simulink model "TrajectoryGeneratorASYNC"  (R2020a)
settings: Solver=FixedStepAuto  StartTime=0.0  StopTime=inf  RelTol=1e-3
model workspace (MAT data in the model file):
  SL_ROS_VariableLengthArrays_MaxSizes.CommonInfo.ArrayTruncateAction = 'EmitWarning'
  SL_ROS_VariableLengthArrays_MaxSizes.MsgTypeMap = containers.Map
  SL_ROS_VariableLengthArrays_MaxSizes.MsgTypeMap.serialization.keys = {}
  SL_ROS_VariableLengthArrays_MaxSizes.MsgTypeMap.serialization.values = {}
  SL_ROS_VariableLengthArrays_MaxSizes.MsgTypeMap.serialization.uniformity = 0
  SL_ROS_VariableLengthArrays_MaxSizes.MsgTypeMap.serialization.keyType = 'char'
  SL_ROS_VariableLengthArrays_MaxSizes.MsgTypeMap.serialization.valueType = 'any'
settings Model: Creator=Lamarre  LastModifiedBy=alexemdesgagne
settings DataIOCC: SaveOutput=off  SaveTime=off
settings OptimizationCC: EnhancedBackFolding=on  PassReuseOutputArgsAs=Individual arguments  ZeroExternalMemoryAtStartup=off  ZeroInternalMemoryAtStartup=off  MaxStackSize=64  OptimizeBlockOrder=speed  DifferentSizesBufferReuse=on  OptimizationCustomize=off  EfficientTunableParamExpr=on
settings DebuggingCC: ParameterTunabilityLossMsg=error  FcnCallInpInsideContextMsg=warning  UnderSpecifiedDimensionMsg=warning
settings HardwareCC: ProdBitPerLong=64  ProdHWDeviceType=Intel->x86-64 (Linux 64)
settings ModelReferenceCC: ModelReferenceNumInstancesAllowed=Single
settings SFSimCC: MATLABDynamicMemAlloc=off
settings RTWCC: SystemTargetFile=ert.tlc  HardwareBoard=Robot Operating System (ROS)  TemplateMakefile=ert_default_tmf  Toolchain=Catkin  BuildConfiguration=Faster Runs  TargetLang=C++
settings CodeAppCC: ForceParamTrailComments=on  IgnoreCustomStorageClasses=off  OperatorAnnotations=on  SimulinkDataObjDesc=on  SFDataObjDesc=on  InsertBlockDesc=on
settings ERTTargetCC: SuppressErrorStatus=on  SupportVariableSizeSignals=on  MultiInstanceErrorCode=Warning  RootIOFormat=Structure reference

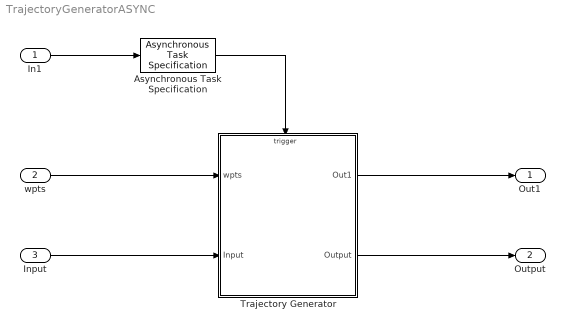
== system TrajectoryGeneratorASYNC ==
  In1 : Inport  OutDataTypeStr=boolean  PortDimensions=1  OutputFunctionCall=on
  wpts : Inport  Port=2  OutDataTypeStr=double  PortDimensions=[20 7]
  Input : Inport  Port=3  OutDataTypeStr=double  PortDimensions=[1 1]
  Asynchronous Task Specification : AsynchronousTaskSpecification
  Trajectory Generator : Subsystem  TreatAsAtomicUnit=on
  Out1 : Outport  OutDataTypeStr=double  PortDimensions=[1000 13]
  Output : Outport  Port=2  OutDataTypeStr=double  PortDimensions=[1 2]
  wires:
  Trajectory Generator/2(Output) -> Output/1
  In1/1 -> Asynchronous Task Specification/1
  Asynchronous Task Specification/1 -> Trajectory Generator/Trigger
  wpts/1 -> Trajectory Generator/1(wpts)
  Trajectory Generator/1(Out1) -> Out1/1
  Input/1 -> Trajectory Generator/2(Input)

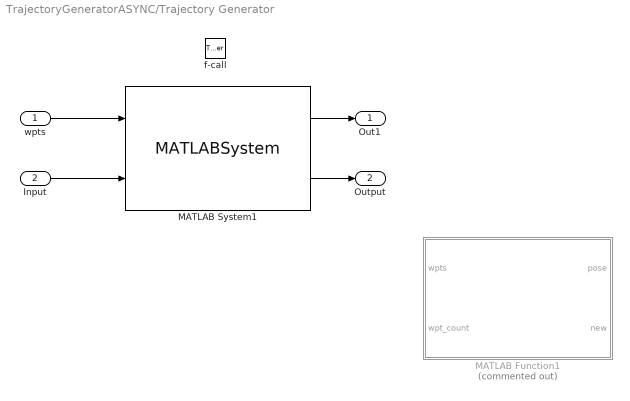
== system TrajectoryGeneratorASYNC/Trajectory Generator ==
  wpts : Inport
  Input : Inport  Port=2
  f-call : TriggerPort  TriggerType=function-call  VariantControl=Variant
  MATLAB Function1 : MATLAB Function  Commented=on  TreatAsAtomicUnit=on
  MATLAB System1 : MATLABSystem  System=TrajectoryGenerator  avanceRapide=1  avancePrecision=0.5  accRapide=0.3  accPrecision=0.1  Ts=0.25  bufferSize=1000  SimulateUsing=Code generation
      mask Type: TrajectoryGenerator
      mask Display:
      | disp('TrajectoryGenerator');
      | port_label('input',1,'wpts');
      | port_label('input',2,'wpt_count');
      | port_label('output',1,'pose');
      | port_label('output',2,'new');
  Out1 : Outport
  Output : Outport  Port=2
  wires:
  wpts/1 -> MATLAB System1/1
  Input/1 -> MATLAB System1/2
  MATLAB System1/1 -> Out1/1
  MATLAB System1/2 -> Output/1

== matlab function TrajectoryGeneratorASYNC/Trajectory Generator/MATLAB Function1 ==
  data: wpts input size=[20 7]; pose output size=[1000 13]; wpt_count input; new output
function [pose, new] = fcn(wpts, wpt_count)
 avanceRapide = 1; % Vitesse Rapide
 avancePrecision = 0.5; % Vtesse Precision

 accRapide = 0.3; % acceleration Rapide
 accPrecision = 0.1; % acceleration Precision
 
 bufferSize=1000; % Taille statique 
 
 Ts=.25;
 
 computeCount=0;
 
  % Implement algorithm. Calculate y as a function of input u and
            % discrete states.
        
            % Initialiser les tableau
            linwpts = wpts(:,1:3);% wpts(1:wpt_count-1,1:3);
            
            
            qwpts = zeros(size(wpts, 1), 4);
            
           
            for k = 1:size(wpts, 1)
                %linwpts(k, 1:3) = wpts(k,1:3);
                qwpts(k, 1:4) = wpts(k,4:7);
            end
            
            for i=wpt_count-1:size(wpts, 1)
                linwpts(i,:) = linwpts(wpt_count-1,:);
                qwpts(i,:) = qwpts(wpt_count-1,:);
            end
            
            quatwpts = quaternion(qwpts);
            
           

            % Gestion des vitesses et des accélérations.
            
            
            % Génération d'un vecteur de temps
            tpts = zeros(size(wpts, 1),1);
            
            for i = 2: wpt_count-1
                dist = norm(wpts(i,1:3) - wpts(i-1,1:3));
                temp = dist / avancePrecision + 2 * (avancePrecision / accRapide);
                tpts(i) = temp + tpts(i-1);
            end
            
            for i=wpt_count : size(tpts,1)
                tpts(i)=tpts(i-1)+.01 ;
            end
                
                
            %tpts = [0,20,40,60,80,95,120,130,150,175,200,230,250,275,300];
            
          
            
            final=tpts(wpt_count-1);
            
            nbPoint=floor(final/Ts);
            
            trajectory = waypointTrajectory(linwpts, tpts,'SampleRate', 1/Ts,'SamplesPerFrame',1, 'Orientation', quatwpts);
            pose=repmat(999,bufferSize, 13);
            

           nbpts=1;
           for i=1 : nbPoint
                    
                   [bufferPose, bufferQuat, bufferVelocity , acc ,bufferAngRate] = trajectory();%, bufferVelocity, bufferAcc, bufferAngRate
                    pose(i, 1:3) = bufferPose;
                    pose(i, 4:7) = compact(bufferQuat);
                    pose(i, 8:10) = bufferVelocity;
                    pose(i, 11:13) = bufferAngRate;
                    nbpts=i;
                  
            end
            computeCount = computeCount + 1;
            new = [computeCount,  nbpts];
            disp("run")
 
end
